simulink model "souk_dual_pipeline_krm"  (R2021a)
settings: Solver=VariableStepAuto  StartTime=0.0  StopTime=10.0  RelTol=1e-3
undefined symbols (not defined in the file): datetime, emio_enet2_tsu_timer_cmp_val_0, posixtime, signal
libraries: xbsIndex_r4 x15746, casper_library_misc x108, casper_library_delays x65, casper_library_reorder x44, xps_library x12
(part 60 of 175)

== system souk_dual_pipeline_krm/p1/synth_input_reorder3/bus_mux ==
  sel : Inport
  d0 : Inport  Port=2
  d1 : Inport  Port=3
  d2 : Inport  Port=4
  d3 : Inport  Port=5
  d4 : Inport  Port=6
  misci : Inport  Port=7
  d_bussify : Subsystem  AncestorBlock=casper_library_flow_control/bus_create  mask(bus_create){inputNum=16}
      mask prompts: inputNum "Number of inputs:"
      mask init:
      | bus_create_init(gcb,...
      |     'inputNum', inputNum);
  dmisc : xbsIndex_r4/Delay  rst=off  infoeditControl=Selection of Reset will increase slice count due to use of real FFs and instead of SRLs  en=off  latency=0  reg_retiming=on  dbl_ovrd=off  block_type=delay
  expand0 : Subsystem  AncestorBlock=casper_library_flow_control/bus_expand  mask(bus_expand){mode=divisions of arbitrary size, outputNum=2, outputWidth=[36;36;36;36;36;36;36;36;36;36;36;36;36;36;36;36], outputBinaryPt=[0  0  0  0  0  0  0  0  0  0  0  0  0  0  0  0], outputArithmeticType=[0  0  0  0  0  0  0  0  0  0  0  0  0  0  0  0], show_format=on, outputToWorkspace=off, variablePrefix=, outputToModelAsWell=on}
      mask prompts: outputNum "Number of outputs:"; outputWidth "Output width:"; outputBinaryPt "Output binary point position:"; outputArithmeticType "Output arithmetic type (ufix=0, fix=1, bool=2):"; show_format "Print format string?"; outputToWorkspace "Output to workspace?"; variablePrefix "Variable name prefix:"; outputToModelAsWell "Output to model as well?"
      mask help:
      | Expands a 'bus' made using a bus_create or Xilinx
      | concat block.
      | The input will be divided into the specified number
      | of outputs with the specified arithmetic types.
      | Divisions are made from most significant bit.
      mask init: same as souk_dual_pipeline_krm/bus_expand
      settings: AttributesFormatString=16 outputs: uf36.0,uf36.0,uf36.0,uf36.0,uf36.0,uf36.0,uf36.0,uf36.0,uf36.0,uf36.0,uf36.0,uf36.0,uf36.0,uf36.0,uf36.0,uf36.0,
      mask TypeOptions mode: divisions of equal size | divisions of arbitrary size
      mask Callback mode: %bus_expand_callback();
      mask Callback outputWidth: %bus_expand_callback();
      mask Callback outputToWorkspace: %bus_expand_callback();
  expand1 : Subsystem  AncestorBlock=casper_library_flow_control/bus_expand  mask(bus_expand){mode=divisions of arbitrary size, outputNum=2, outputWidth=[36;36;36;36;36;36;36;36;36;36;36;36;36;36;36;36], outputBinaryPt=[0  0  0  0  0  0  0  0  0  0  0  0  0  0  0  0], outputArithmeticType=[0  0  0  0  0  0  0  0  0  0  0  0  0  0  0  0], show_format=on, outputToWorkspace=off, variablePrefix=, outputToModelAsWell=on}
      mask prompts: outputNum "Number of outputs:"; outputWidth "Output width:"; outputBinaryPt "Output binary point position:"; outputArithmeticType "Output arithmetic type (ufix=0, fix=1, bool=2):"; show_format "Print format string?"; outputToWorkspace "Output to workspace?"; variablePrefix "Variable name prefix:"; outputToModelAsWell "Output to model as well?"
      mask help:
      | Expands a 'bus' made using a bus_create or Xilinx
      | concat block.
      | The input will be divided into the specified number
      | of outputs with the specified arithmetic types.
      | Divisions are made from most significant bit.
      mask init: same as souk_dual_pipeline_krm/bus_expand
      settings: AttributesFormatString=16 outputs: uf36.0,uf36.0,uf36.0,uf36.0,uf36.0,uf36.0,uf36.0,uf36.0,uf36.0,uf36.0,uf36.0,uf36.0,uf36.0,uf36.0,uf36.0,uf36.0,
      mask TypeOptions mode: divisions of equal size | divisions of arbitrary size
      mask Callback mode: %bus_expand_callback();
      mask Callback outputWidth: %bus_expand_callback();
      mask Callback outputToWorkspace: %bus_expand_callback();
  expand2 : Subsystem  AncestorBlock=casper_library_flow_control/bus_expand  mask(bus_expand){mode=divisions of arbitrary size, outputNum=2, outputWidth=[36;36;36;36;36;36;36;36;36;36;36;36;36;36;36;36], outputBinaryPt=[0  0  0  0  0  0  0  0  0  0  0  0  0  0  0  0], outputArithmeticType=[0  0  0  0  0  0  0  0  0  0  0  0  0  0  0  0], show_format=on, outputToWorkspace=off, variablePrefix=, outputToModelAsWell=on}
      mask prompts: outputNum "Number of outputs:"; outputWidth "Output width:"; outputBinaryPt "Output binary point position:"; outputArithmeticType "Output arithmetic type (ufix=0, fix=1, bool=2):"; show_format "Print format string?"; outputToWorkspace "Output to workspace?"; variablePrefix "Variable name prefix:"; outputToModelAsWell "Output to model as well?"
      mask help:
      | Expands a 'bus' made using a bus_create or Xilinx
      | concat block.
      | The input will be divided into the specified number
      | of outputs with the specified arithmetic types.
      | Divisions are made from most significant bit.
      mask init: same as souk_dual_pipeline_krm/bus_expand
      settings: AttributesFormatString=16 outputs: uf36.0,uf36.0,uf36.0,uf36.0,uf36.0,uf36.0,uf36.0,uf36.0,uf36.0,uf36.0,uf36.0,uf36.0,uf36.0,uf36.0,uf36.0,uf36.0,
      mask TypeOptions mode: divisions of equal size | divisions of arbitrary size
      mask Callback mode: %bus_expand_callback();
      mask Callback outputWidth: %bus_expand_callback();
      mask Callback outputToWorkspace: %bus_expand_callback();
  expand3 : Subsystem  AncestorBlock=casper_library_flow_control/bus_expand  mask(bus_expand){mode=divisions of arbitrary size, outputNum=2, outputWidth=[36;36;36;36;36;36;36;36;36;36;36;36;36;36;36;36], outputBinaryPt=[0  0  0  0  0  0  0  0  0  0  0  0  0  0  0  0], outputArithmeticType=[0  0  0  0  0  0  0  0  0  0  0  0  0  0  0  0], show_format=on, outputToWorkspace=off, variablePrefix=, outputToModelAsWell=on}
      mask prompts: outputNum "Number of outputs:"; outputWidth "Output width:"; outputBinaryPt "Output binary point position:"; outputArithmeticType "Output arithmetic type (ufix=0, fix=1, bool=2):"; show_format "Print format string?"; outputToWorkspace "Output to workspace?"; variablePrefix "Variable name prefix:"; outputToModelAsWell "Output to model as well?"
      mask help:
      | Expands a 'bus' made using a bus_create or Xilinx
      | concat block.
      | The input will be divided into the specified number
      | of outputs with the specified arithmetic types.
      | Divisions are made from most significant bit.
      mask init: same as souk_dual_pipeline_krm/bus_expand
      settings: AttributesFormatString=16 outputs: uf36.0,uf36.0,uf36.0,uf36.0,uf36.0,uf36.0,uf36.0,uf36.0,uf36.0,uf36.0,uf36.0,uf36.0,uf36.0,uf36.0,uf36.0,uf36.0,
      mask TypeOptions mode: divisions of equal size | divisions of arbitrary size
      mask Callback mode: %bus_expand_callback();
      mask Callback outputWidth: %bus_expand_callback();
      mask Callback outputToWorkspace: %bus_expand_callback();
  expand4 : Subsystem  AncestorBlock=casper_library_flow_control/bus_expand  mask(bus_expand){mode=divisions of arbitrary size, outputNum=2, outputWidth=[36;36;36;36;36;36;36;36;36;36;36;36;36;36;36;36], outputBinaryPt=[0  0  0  0  0  0  0  0  0  0  0  0  0  0  0  0], outputArithmeticType=[0  0  0  0  0  0  0  0  0  0  0  0  0  0  0  0], show_format=on, outputToWorkspace=off, variablePrefix=, outputToModelAsWell=on}
      mask prompts: outputNum "Number of outputs:"; outputWidth "Output width:"; outputBinaryPt "Output binary point position:"; outputArithmeticType "Output arithmetic type (ufix=0, fix=1, bool=2):"; show_format "Print format string?"; outputToWorkspace "Output to workspace?"; variablePrefix "Variable name prefix:"; outputToModelAsWell "Output to model as well?"
      mask help:
      | Expands a 'bus' made using a bus_create or Xilinx
      | concat block.
      | The input will be divided into the specified number
      | of outputs with the specified arithmetic types.
      | Divisions are made from most significant bit.
      mask init: same as souk_dual_pipeline_krm/bus_expand
      settings: AttributesFormatString=16 outputs: uf36.0,uf36.0,uf36.0,uf36.0,uf36.0,uf36.0,uf36.0,uf36.0,uf36.0,uf36.0,uf36.0,uf36.0,uf36.0,uf36.0,uf36.0,uf36.0,
      mask TypeOptions mode: divisions of equal size | divisions of arbitrary size
      mask Callback mode: %bus_expand_callback();
      mask Callback outputWidth: %bus_expand_callback();
      mask Callback outputToWorkspace: %bus_expand_callback();
  mux{0..15} (16 alike) : xbsIndex_r4/Mux  inputs=5  en=off  latency=0  precision=Full  arith_type=Unsigned  n_bits=16  bin_pt=14  quantization=Truncate  overflow=Wrap  dbl_ovrd=off  block_type=mux
  sel_expand : Subsystem  AncestorBlock=casper_library_flow_control/bus_expand  mask(bus_expand){mode=divisions of equal size, outputNum=16, outputWidth=3, outputBinaryPt=0, outputArithmeticType=0, show_format=on, outputToWorkspace=off, variablePrefix=, outputToModelAsWell=on}
      mask prompts: outputNum "Number of outputs:"; outputWidth "Output width:"; outputBinaryPt "Output binary point position:"; outputArithmeticType "Output arithmetic type (ufix=0, fix=1, bool=2):"; show_format "Print format string?"; outputToWorkspace "Output to workspace?"; variablePrefix "Variable name prefix:"; outputToModelAsWell "Output to model as well?"
      mask help:
      | Expands a 'bus' made using a bus_create or Xilinx
      | concat block.
      | The input will be divided into the specified number
      | of outputs with the specified arithmetic types.
      | Divisions are made from most significant bit.
      mask init: same as souk_dual_pipeline_krm/bus_expand
      settings: AttributesFormatString=16 outputs: uf3.0,uf3.0,uf3.0,uf3.0,uf3.0,uf3.0,uf3.0,uf3.0,uf3.0,uf3.0,uf3.0,uf3.0,uf3.0,uf3.0,uf3.0,uf3.0,
      mask TypeOptions mode: divisions of equal size | divisions of arbitrary size
      mask Callback mode: %bus_expand_callback();
      mask Callback outputWidth: %bus_expand_callback();
      mask Callback outputToWorkspace: %bus_expand_callback();
  out : Outport
  misco : Outport  Port=2
  wires:
  sel/1 -> sel_expand/1(bus_in)
  d0/1 -> expand0/1(bus_in)
  d1/1 -> expand1/1(bus_in)
  d2/1 -> expand2/1(bus_in)
  d3/1 -> expand3/1(bus_in)
  d4/1 -> expand4/1(bus_in)
  sel_expand/1(msb_out16) -> mux0/1
  expand0/1(msb_out16) -> mux0/2
  expand1/1(msb_out16) -> mux0/3
  expand2/1(msb_out16) -> mux0/4
  expand3/1(msb_out16) -> mux0/5
  expand4/1(msb_out16) -> mux0/6
  sel_expand/2(out15) -> mux1/1
  expand0/2(out15) -> mux1/2
  expand1/2(out15) -> mux1/3
  expand2/2(out15) -> mux1/4
  expand3/2(out15) -> mux1/5
  expand4/2(out15) -> mux1/6
  sel_expand/3(out14) -> mux2/1
  expand0/3(out14) -> mux2/2
  expand1/3(out14) -> mux2/3
  expand2/3(out14) -> mux2/4
  expand3/3(out14) -> mux2/5
  expand4/3(out14) -> mux2/6
  sel_expand/4(out13) -> mux3/1
  expand0/4(out13) -> mux3/2
  expand1/4(out13) -> mux3/3
  expand2/4(out13) -> mux3/4
  expand3/4(out13) -> mux3/5
  expand4/4(out13) -> mux3/6
  sel_expand/5(out12) -> mux4/1
  expand0/5(out12) -> mux4/2
  expand1/5(out12) -> mux4/3
  expand2/5(out12) -> mux4/4
  expand3/5(out12) -> mux4/5
  expand4/5(out12) -> mux4/6
  sel_expand/6(out11) -> mux5/1
  expand0/6(out11) -> mux5/2
  expand1/6(out11) -> mux5/3
  expand2/6(out11) -> mux5/4
  expand3/6(out11) -> mux5/5
  expand4/6(out11) -> mux5/6
  sel_expand/7(out10) -> mux6/1
  expand0/7(out10) -> mux6/2
  expand1/7(out10) -> mux6/3
  expand2/7(out10) -> mux6/4
  expand3/7(out10) -> mux6/5
  expand4/7(out10) -> mux6/6
  sel_expand/8(out9) -> mux7/1
  expand0/8(out9) -> mux7/2
  expand1/8(out9) -> mux7/3
  expand2/8(out9) -> mux7/4
  expand3/8(out9) -> mux7/5
  expand4/8(out9) -> mux7/6
  sel_expand/9(out8) -> mux8/1
  expand0/9(out8) -> mux8/2
  expand1/9(out8) -> mux8/3
  expand2/9(out8) -> mux8/4
  expand3/9(out8) -> mux8/5
  expand4/9(out8) -> mux8/6
  sel_expand/10(out7) -> mux9/1
  expand0/10(out7) -> mux9/2
  expand1/10(out7) -> mux9/3
  expand2/10(out7) -> mux9/4
  expand3/10(out7) -> mux9/5
  expand4/10(out7) -> mux9/6
  sel_expand/11(out6) -> mux10/1
  expand0/11(out6) -> mux10/2
  expand1/11(out6) -> mux10/3
  expand2/11(out6) -> mux10/4
  expand3/11(out6) -> mux10/5
  expand4/11(out6) -> mux10/6
  sel_expand/12(out5) -> mux11/1
  expand0/12(out5) -> mux11/2
  expand1/12(out5) -> mux11/3
  expand2/12(out5) -> mux11/4
  expand3/12(out5) -> mux11/5
  expand4/12(out5) -> mux11/6
  sel_expand/13(out4) -> mux12/1
  expand0/13(out4) -> mux12/2
  expand1/13(out4) -> mux12/3
  expand2/13(out4) -> mux12/4
  expand3/13(out4) -> mux12/5
  expand4/13(out4) -> mux12/6
  sel_expand/14(out3) -> mux13/1
  expand0/14(out3) -> mux13/2
  expand1/14(out3) -> mux13/3
  expand2/14(out3) -> mux13/4
  expand3/14(out3) -> mux13/5
  expand4/14(out3) -> mux13/6
  sel_expand/15(out2) -> mux14/1
  expand0/15(out2) -> mux14/2
  expand1/15(out2) -> mux14/3
  expand2/15(out2) -> mux14/4
  expand3/15(out2) -> mux14/5
  expand4/15(out2) -> mux14/6
  sel_expand/16(lsb_out1) -> mux15/1
  expand0/16(lsb_out1) -> mux15/2
  expand1/16(lsb_out1) -> mux15/3
  expand2/16(lsb_out1) -> mux15/4
  expand3/16(lsb_out1) -> mux15/5
  expand4/16(lsb_out1) -> mux15/6
  misci/1 -> dmisc/1
  mux0/1 -> d_bussify/1(in1)
  mux1/1 -> d_bussify/2(in2)
  mux2/1 -> d_bussify/3(in3)
  mux3/1 -> d_bussify/4(in4)
  mux4/1 -> d_bussify/5(in5)
  mux5/1 -> d_bussify/6(in6)
  mux6/1 -> d_bussify/7(in7)
  mux7/1 -> d_bussify/8(in8)
  mux8/1 -> d_bussify/9(in9)
  mux9/1 -> d_bussify/10(in10)
  mux10/1 -> d_bussify/11(in11)
  mux11/1 -> d_bussify/12(in12)
  mux12/1 -> d_bussify/13(in13)
  mux13/1 -> d_bussify/14(in14)
  mux14/1 -> d_bussify/15(in15)
  mux15/1 -> d_bussify/16(in16)
  d_bussify/1(bus_out) -> out/1
  dmisc/1 -> misco/1

== system souk_dual_pipeline_krm/p1/synth_input_reorder3/bus_replicate ==
  in : Inport
  bussify : Subsystem  AncestorBlock=casper_library_flow_control/bus_create  mask(bus_create){inputNum=16}
      mask prompts: inputNum "Number of inputs:"
      mask init:
      | bus_create_init(gcb,...
      |     'inputNum', inputNum);
  out : Outport
  wires:
  in/1 -> bussify/1(in1), bussify/2(in2), bussify/3(in3), bussify/4(in4), bussify/5(in5), bussify/6(in6), bussify/7(in7), bussify/8(in8), bussify/9(in9), bussify/10(in10), bussify/11(in11), bussify/12(in12), bussify/13(in13), bussify/14(in14), bussify/15(in15), bussify/16(in16)
  bussify/1(bus_out) -> out/1

== system souk_dual_pipeline_krm/p1/synth_input_reorder3/bus_replicate1 ==
  in : Inport
  bussify : Subsystem  AncestorBlock=casper_library_flow_control/bus_create  mask(bus_create){inputNum=16}
      mask prompts: inputNum "Number of inputs:"
      mask init:
      | bus_create_init(gcb,...
      |     'inputNum', inputNum);
  out : Outport
  wires:
  bussify/1(bus_out) -> out/1
  in/1 -> bussify/16(in16), bussify/15(in15), bussify/14(in14), bussify/13(in13), bussify/12(in12), bussify/11(in11), bussify/10(in10), bussify/9(in9), bussify/8(in8), bussify/7(in7), bussify/6(in6), bussify/5(in5), bussify/4(in4), bussify/3(in3), bussify/2(in2), bussify/1(in1)

== system souk_dual_pipeline_krm/p1/synth_input_reorder3/bus_replicate2 ==
  in : Inport
  bussify : Subsystem  AncestorBlock=casper_library_flow_control/bus_create  mask(bus_create){inputNum=16}
      mask prompts: inputNum "Number of inputs:"
      mask init:
      | bus_create_init(gcb,...
      |     'inputNum', inputNum);
  out : Outport
  wires:
  in/1 -> bussify/1(in1), bussify/2(in2), bussify/3(in3), bussify/4(in4), bussify/5(in5), bussify/6(in6), bussify/7(in7), bussify/8(in8), bussify/9(in9), bussify/10(in10), bussify/11(in11), bussify/12(in12), bussify/13(in13), bussify/14(in14), bussify/15(in15), bussify/16(in16)
  bussify/1(bus_out) -> out/1

== system souk_dual_pipeline_krm/p1/synth_input_reorder3/bus_replicate3 ==
  in : Inport
  bussify : Subsystem  AncestorBlock=casper_library_flow_control/bus_create  mask(bus_create){inputNum=16}
      mask prompts: inputNum "Number of inputs:"
      mask init:
      | bus_create_init(gcb,...
      |     'inputNum', inputNum);
  out : Outport
  wires:
  bussify/1(bus_out) -> out/1
  in/1 -> bussify/16(in16), bussify/15(in15), bussify/14(in14), bussify/13(in13), bussify/12(in12), bussify/11(in11), bussify/10(in10), bussify/9(in9), bussify/8(in8), bussify/7(in7), bussify/6(in6), bussify/5(in5), bussify/4(in4), bussify/3(in3), bussify/2(in2), bussify/1(in1)

== system souk_dual_pipeline_krm/p1/synth_input_reorder3/map0 ==
  sync : Inport
  din0 : Inport  Port=2
  Constant1 : xbsIndex_r4/Constant  const=1.0  gui_display_data_type=Boolean  arith_type=Boolean  n_bits=16  bin_pt=14  preci_type=Single  exp_width=8  frac_width=24  explicit_period=on  period=1  equ=P=C  opselect=C  inp2=PCIN>>17  opr=+  inp1=P  carry=CIN  dbl_ovrd=off  block_type=constant
  reord : Subsystem  AncestorBlock=casper_library_reorder/reorder  mask(reorder){map=[2^(serial_chan_bits)-1:-1:0], n_bits=0, n_inputs=1, bram_latency=2, map_latency=1, fanout_latency=0, double_buffer=1, bram_map=off, software_controlled=on, use_control_fanout=on, hide_latency=on}
      mask prompts: map "Output Order:"; n_bits "Data width in"; n_inputs "Number of inputs"; bram_latency "BRAM Latency"; map_latency "Map Latency"; fanout_latency "Fanout latency"; double_buffer "Double Buffer"; bram_map "Use BlockRAM for Map"; software_controlled "Use runtime software control"; use_control_fanout "Control fanout of control to multiple iniputs"; hide_latency "EXPERIMENTAL: Hide control latency"
      mask init: same as souk_dual_pipeline_krm/p0/chan_select/2
      settings: AttributesFormatString=order=2
      mask Help: eval('xlWeb(''http://casper.berkeley.edu/wiki/Reorder'')')
  sync_out : Outport
  dout : Outport  Port=2
  wires:
  reord/3(dout0) -> dout/1
  din0/1 -> reord/3(din0)
  reord/1(sync_out) -> sync_out/1
  Constant1/1 -> reord/2(en)
  sync/1 -> reord/1(sync)
  reord/2(valid) -> ?

== system souk_dual_pipeline_krm/p1/synth_input_reorder3/map1 ==
  sync : Inport
  din0 : Inport  Port=2
  Constant1 : xbsIndex_r4/Constant  const=1.0  gui_display_data_type=Boolean  arith_type=Boolean  n_bits=16  bin_pt=14  preci_type=Single  exp_width=8  frac_width=24  explicit_period=on  period=1  equ=P=C  opselect=C  inp2=PCIN>>17  opr=+  inp1=P  carry=CIN  dbl_ovrd=off  block_type=constant
  reord : Subsystem  AncestorBlock=casper_library_reorder/reorder  mask(reorder){map=[2^(serial_chan_bits)-1:-1:0], n_bits=0, n_inputs=1, bram_latency=2, map_latency=1, fanout_latency=0, double_buffer=1, bram_map=off, software_controlled=on, use_control_fanout=on, hide_latency=on}
      mask prompts: map "Output Order:"; n_bits "Data width in"; n_inputs "Number of inputs"; bram_latency "BRAM Latency"; map_latency "Map Latency"; fanout_latency "Fanout latency"; double_buffer "Double Buffer"; bram_map "Use BlockRAM for Map"; software_controlled "Use runtime software control"; use_control_fanout "Control fanout of control to multiple iniputs"; hide_latency "EXPERIMENTAL: Hide control latency"
      mask init: same as souk_dual_pipeline_krm/p0/chan_select/2
      settings: AttributesFormatString=order=2
      mask Help: eval('xlWeb(''http://casper.berkeley.edu/wiki/Reorder'')')
  sync_out : Outport
  dout : Outport  Port=2
  wires:
  reord/2(valid) -> ?
  sync/1 -> reord/1(sync)
  Constant1/1 -> reord/2(en)
  reord/1(sync_out) -> sync_out/1
  din0/1 -> reord/3(din0)
  reord/3(dout0) -> dout/1

== system souk_dual_pipeline_krm/p1/synth_input_reorder3/map10 ==
  sync : Inport
  din0 : Inport  Port=2
  Constant1 : xbsIndex_r4/Constant  const=1.0  gui_display_data_type=Boolean  arith_type=Boolean  n_bits=16  bin_pt=14  preci_type=Single  exp_width=8  frac_width=24  explicit_period=on  period=1  equ=P=C  opselect=C  inp2=PCIN>>17  opr=+  inp1=P  carry=CIN  dbl_ovrd=off  block_type=constant
  reord : Subsystem  AncestorBlock=casper_library_reorder/reorder  mask(reorder){map=[2^(serial_chan_bits)-1:-1:0], n_bits=0, n_inputs=1, bram_latency=2, map_latency=1, fanout_latency=0, double_buffer=1, bram_map=off, software_controlled=on, use_control_fanout=on, hide_latency=on}
      mask prompts: map "Output Order:"; n_bits "Data width in"; n_inputs "Number of inputs"; bram_latency "BRAM Latency"; map_latency "Map Latency"; fanout_latency "Fanout latency"; double_buffer "Double Buffer"; bram_map "Use BlockRAM for Map"; software_controlled "Use runtime software control"; use_control_fanout "Control fanout of control to multiple iniputs"; hide_latency "EXPERIMENTAL: Hide control latency"
      mask init: same as souk_dual_pipeline_krm/p0/chan_select/2
      settings: AttributesFormatString=order=2
      mask Help: eval('xlWeb(''http://casper.berkeley.edu/wiki/Reorder'')')
  sync_out : Outport
  dout : Outport  Port=2
  wires:
  reord/3(dout0) -> dout/1
  din0/1 -> reord/3(din0)
  reord/1(sync_out) -> sync_out/1
  Constant1/1 -> reord/2(en)
  sync/1 -> reord/1(sync)
  reord/2(valid) -> ?

== system souk_dual_pipeline_krm/p1/synth_input_reorder3/map11 ==
  sync : Inport
  din0 : Inport  Port=2
  Constant1 : xbsIndex_r4/Constant  const=1.0  gui_display_data_type=Boolean  arith_type=Boolean  n_bits=16  bin_pt=14  preci_type=Single  exp_width=8  frac_width=24  explicit_period=on  period=1  equ=P=C  opselect=C  inp2=PCIN>>17  opr=+  inp1=P  carry=CIN  dbl_ovrd=off  block_type=constant
  reord : Subsystem  AncestorBlock=casper_library_reorder/reorder  mask(reorder){map=[2^(serial_chan_bits)-1:-1:0], n_bits=0, n_inputs=1, bram_latency=2, map_latency=1, fanout_latency=0, double_buffer=1, bram_map=off, software_controlled=on, use_control_fanout=on, hide_latency=on}
      mask prompts: map "Output Order:"; n_bits "Data width in"; n_inputs "Number of inputs"; bram_latency "BRAM Latency"; map_latency "Map Latency"; fanout_latency "Fanout latency"; double_buffer "Double Buffer"; bram_map "Use BlockRAM for Map"; software_controlled "Use runtime software control"; use_control_fanout "Control fanout of control to multiple iniputs"; hide_latency "EXPERIMENTAL: Hide control latency"
      mask init: same as souk_dual_pipeline_krm/p0/chan_select/2
      settings: AttributesFormatString=order=2
      mask Help: eval('xlWeb(''http://casper.berkeley.edu/wiki/Reorder'')')
  sync_out : Outport
  dout : Outport  Port=2
  wires:
  reord/2(valid) -> ?
  sync/1 -> reord/1(sync)
  Constant1/1 -> reord/2(en)
  reord/1(sync_out) -> sync_out/1
  din0/1 -> reord/3(din0)
  reord/3(dout0) -> dout/1

== system souk_dual_pipeline_krm/p1/synth_input_reorder3/map12 ==
  sync : Inport
  din0 : Inport  Port=2
  Constant1 : xbsIndex_r4/Constant  const=1.0  gui_display_data_type=Boolean  arith_type=Boolean  n_bits=16  bin_pt=14  preci_type=Single  exp_width=8  frac_width=24  explicit_period=on  period=1  equ=P=C  opselect=C  inp2=PCIN>>17  opr=+  inp1=P  carry=CIN  dbl_ovrd=off  block_type=constant
  reord : Subsystem  AncestorBlock=casper_library_reorder/reorder  mask(reorder){map=[2^(serial_chan_bits)-1:-1:0], n_bits=0, n_inputs=1, bram_latency=2, map_latency=1, fanout_latency=0, double_buffer=1, bram_map=off, software_controlled=on, use_control_fanout=on, hide_latency=on}
      mask prompts: map "Output Order:"; n_bits "Data width in"; n_inputs "Number of inputs"; bram_latency "BRAM Latency"; map_latency "Map Latency"; fanout_latency "Fanout latency"; double_buffer "Double Buffer"; bram_map "Use BlockRAM for Map"; software_controlled "Use runtime software control"; use_control_fanout "Control fanout of control to multiple iniputs"; hide_latency "EXPERIMENTAL: Hide control latency"
      mask init: same as souk_dual_pipeline_krm/p0/chan_select/2
      settings: AttributesFormatString=order=2
      mask Help: eval('xlWeb(''http://casper.berkeley.edu/wiki/Reorder'')')
  sync_out : Outport
  dout : Outport  Port=2
  wires:
  reord/3(dout0) -> dout/1
  din0/1 -> reord/3(din0)
  reord/1(sync_out) -> sync_out/1
  Constant1/1 -> reord/2(en)
  sync/1 -> reord/1(sync)
  reord/2(valid) -> ?

== system souk_dual_pipeline_krm/p1/synth_input_reorder3/map13 ==
  sync : Inport
  din0 : Inport  Port=2
  Constant1 : xbsIndex_r4/Constant  const=1.0  gui_display_data_type=Boolean  arith_type=Boolean  n_bits=16  bin_pt=14  preci_type=Single  exp_width=8  frac_width=24  explicit_period=on  period=1  equ=P=C  opselect=C  inp2=PCIN>>17  opr=+  inp1=P  carry=CIN  dbl_ovrd=off  block_type=constant
  reord : Subsystem  AncestorBlock=casper_library_reorder/reorder  mask(reorder){map=[2^(serial_chan_bits)-1:-1:0], n_bits=0, n_inputs=1, bram_latency=2, map_latency=1, fanout_latency=0, double_buffer=1, bram_map=off, software_controlled=on, use_control_fanout=on, hide_latency=on}
      mask prompts: map "Output Order:"; n_bits "Data width in"; n_inputs "Number of inputs"; bram_latency "BRAM Latency"; map_latency "Map Latency"; fanout_latency "Fanout latency"; double_buffer "Double Buffer"; bram_map "Use BlockRAM for Map"; software_controlled "Use runtime software control"; use_control_fanout "Control fanout of control to multiple iniputs"; hide_latency "EXPERIMENTAL: Hide control latency"
      mask init: same as souk_dual_pipeline_krm/p0/chan_select/2
      settings: AttributesFormatString=order=2
      mask Help: eval('xlWeb(''http://casper.berkeley.edu/wiki/Reorder'')')
  sync_out : Outport
  dout : Outport  Port=2
  wires:
  reord/2(valid) -> ?
  sync/1 -> reord/1(sync)
  Constant1/1 -> reord/2(en)
  reord/1(sync_out) -> sync_out/1
  din0/1 -> reord/3(din0)
  reord/3(dout0) -> dout/1

== system souk_dual_pipeline_krm/p1/synth_input_reorder3/map14 ==
  sync : Inport
  din0 : Inport  Port=2
  Constant1 : xbsIndex_r4/Constant  const=1.0  gui_display_data_type=Boolean  arith_type=Boolean  n_bits=16  bin_pt=14  preci_type=Single  exp_width=8  frac_width=24  explicit_period=on  period=1  equ=P=C  opselect=C  inp2=PCIN>>17  opr=+  inp1=P  carry=CIN  dbl_ovrd=off  block_type=constant
  reord : Subsystem  AncestorBlock=casper_library_reorder/reorder  mask(reorder){map=[2^(serial_chan_bits)-1:-1:0], n_bits=0, n_inputs=1, bram_latency=2, map_latency=1, fanout_latency=0, double_buffer=1, bram_map=off, software_controlled=on, use_control_fanout=on, hide_latency=on}
      mask prompts: map "Output Order:"; n_bits "Data width in"; n_inputs "Number of inputs"; bram_latency "BRAM Latency"; map_latency "Map Latency"; fanout_latency "Fanout latency"; double_buffer "Double Buffer"; bram_map "Use BlockRAM for Map"; software_controlled "Use runtime software control"; use_control_fanout "Control fanout of control to multiple iniputs"; hide_latency "EXPERIMENTAL: Hide control latency"
      mask init: same as souk_dual_pipeline_krm/p0/chan_select/2
      settings: AttributesFormatString=order=2
      mask Help: eval('xlWeb(''http://casper.berkeley.edu/wiki/Reorder'')')
  sync_out : Outport
  dout : Outport  Port=2
  wires:
  reord/2(valid) -> ?
  sync/1 -> reord/1(sync)
  Constant1/1 -> reord/2(en)
  reord/1(sync_out) -> sync_out/1
  din0/1 -> reord/3(din0)
  reord/3(dout0) -> dout/1

== system souk_dual_pipeline_krm/p1/synth_input_reorder3/map15 ==
  sync : Inport
  din0 : Inport  Port=2
  Constant1 : xbsIndex_r4/Constant  const=1.0  gui_display_data_type=Boolean  arith_type=Boolean  n_bits=16  bin_pt=14  preci_type=Single  exp_width=8  frac_width=24  explicit_period=on  period=1  equ=P=C  opselect=C  inp2=PCIN>>17  opr=+  inp1=P  carry=CIN  dbl_ovrd=off  block_type=constant
  reord : Subsystem  AncestorBlock=casper_library_reorder/reorder  mask(reorder){map=[2^(serial_chan_bits)-1:-1:0], n_bits=0, n_inputs=1, bram_latency=2, map_latency=1, fanout_latency=0, double_buffer=1, bram_map=off, software_controlled=on, use_control_fanout=on, hide_latency=on}
      mask prompts: map "Output Order:"; n_bits "Data width in"; n_inputs "Number of inputs"; bram_latency "BRAM Latency"; map_latency "Map Latency"; fanout_latency "Fanout latency"; double_buffer "Double Buffer"; bram_map "Use BlockRAM for Map"; software_controlled "Use runtime software control"; use_control_fanout "Control fanout of control to multiple iniputs"; hide_latency "EXPERIMENTAL: Hide control latency"
      mask init: same as souk_dual_pipeline_krm/p0/chan_select/2
      settings: AttributesFormatString=order=2
      mask Help: eval('xlWeb(''http://casper.berkeley.edu/wiki/Reorder'')')
  sync_out : Outport
  dout : Outport  Port=2
  wires:
  reord/3(dout0) -> dout/1
  din0/1 -> reord/3(din0)
  reord/1(sync_out) -> sync_out/1
  Constant1/1 -> reord/2(en)
  sync/1 -> reord/1(sync)
  reord/2(valid) -> ?

== system souk_dual_pipeline_krm/p1/synth_input_reorder3/map2 ==
  sync : Inport
  din0 : Inport  Port=2
  Constant1 : xbsIndex_r4/Constant  const=1.0  gui_display_data_type=Boolean  arith_type=Boolean  n_bits=16  bin_pt=14  preci_type=Single  exp_width=8  frac_width=24  explicit_period=on  period=1  equ=P=C  opselect=C  inp2=PCIN>>17  opr=+  inp1=P  carry=CIN  dbl_ovrd=off  block_type=constant
  reord : Subsystem  AncestorBlock=casper_library_reorder/reorder  mask(reorder){map=[2^(serial_chan_bits)-1:-1:0], n_bits=0, n_inputs=1, bram_latency=2, map_latency=1, fanout_latency=0, double_buffer=1, bram_map=off, software_controlled=on, use_control_fanout=on, hide_latency=on}
      mask prompts: map "Output Order:"; n_bits "Data width in"; n_inputs "Number of inputs"; bram_latency "BRAM Latency"; map_latency "Map Latency"; fanout_latency "Fanout latency"; double_buffer "Double Buffer"; bram_map "Use BlockRAM for Map"; software_controlled "Use runtime software control"; use_control_fanout "Control fanout of control to multiple iniputs"; hide_latency "EXPERIMENTAL: Hide control latency"
      mask init: same as souk_dual_pipeline_krm/p0/chan_select/2
      settings: AttributesFormatString=order=2
      mask Help: eval('xlWeb(''http://casper.berkeley.edu/wiki/Reorder'')')
  sync_out : Outport
  dout : Outport  Port=2
  wires:
  reord/2(valid) -> ?
  sync/1 -> reord/1(sync)
  Constant1/1 -> reord/2(en)
  reord/1(sync_out) -> sync_out/1
  din0/1 -> reord/3(din0)
  reord/3(dout0) -> dout/1

== system souk_dual_pipeline_krm/p1/synth_input_reorder3/map3 ==
  sync : Inport
  din0 : Inport  Port=2
  Constant1 : xbsIndex_r4/Constant  const=1.0  gui_display_data_type=Boolean  arith_type=Boolean  n_bits=16  bin_pt=14  preci_type=Single  exp_width=8  frac_width=24  explicit_period=on  period=1  equ=P=C  opselect=C  inp2=PCIN>>17  opr=+  inp1=P  carry=CIN  dbl_ovrd=off  block_type=constant
  reord : Subsystem  AncestorBlock=casper_library_reorder/reorder  mask(reorder){map=[2^(serial_chan_bits)-1:-1:0], n_bits=0, n_inputs=1, bram_latency=2, map_latency=1, fanout_latency=0, double_buffer=1, bram_map=off, software_controlled=on, use_control_fanout=on, hide_latency=on}
      mask prompts: map "Output Order:"; n_bits "Data width in"; n_inputs "Number of inputs"; bram_latency "BRAM Latency"; map_latency "Map Latency"; fanout_latency "Fanout latency"; double_buffer "Double Buffer"; bram_map "Use BlockRAM for Map"; software_controlled "Use runtime software control"; use_control_fanout "Control fanout of control to multiple iniputs"; hide_latency "EXPERIMENTAL: Hide control latency"
      mask init: same as souk_dual_pipeline_krm/p0/chan_select/2
      settings: AttributesFormatString=order=2
      mask Help: eval('xlWeb(''http://casper.berkeley.edu/wiki/Reorder'')')
  sync_out : Outport
  dout : Outport  Port=2
  wires:
  reord/3(dout0) -> dout/1
  din0/1 -> reord/3(din0)
  reord/1(sync_out) -> sync_out/1
  Constant1/1 -> reord/2(en)
  sync/1 -> reord/1(sync)
  reord/2(valid) -> ?

== system souk_dual_pipeline_krm/p1/synth_input_reorder3/map4 ==
  sync : Inport
  din0 : Inport  Port=2
  Constant1 : xbsIndex_r4/Constant  const=1.0  gui_display_data_type=Boolean  arith_type=Boolean  n_bits=16  bin_pt=14  preci_type=Single  exp_width=8  frac_width=24  explicit_period=on  period=1  equ=P=C  opselect=C  inp2=PCIN>>17  opr=+  inp1=P  carry=CIN  dbl_ovrd=off  block_type=constant
  reord : Subsystem  AncestorBlock=casper_library_reorder/reorder  mask(reorder){map=[2^(serial_chan_bits)-1:-1:0], n_bits=0, n_inputs=1, bram_latency=2, map_latency=1, fanout_latency=0, double_buffer=1, bram_map=off, software_controlled=on, use_control_fanout=on, hide_latency=on}
      mask prompts: map "Output Order:"; n_bits "Data width in"; n_inputs "Number of inputs"; bram_latency "BRAM Latency"; map_latency "Map Latency"; fanout_latency "Fanout latency"; double_buffer "Double Buffer"; bram_map "Use BlockRAM for Map"; software_controlled "Use runtime software control"; use_control_fanout "Control fanout of control to multiple iniputs"; hide_latency "EXPERIMENTAL: Hide control latency"
      mask init: same as souk_dual_pipeline_krm/p0/chan_select/2
      settings: AttributesFormatString=order=2
      mask Help: eval('xlWeb(''http://casper.berkeley.edu/wiki/Reorder'')')
  sync_out : Outport
  dout : Outport  Port=2
  wires:
  reord/2(valid) -> ?
  sync/1 -> reord/1(sync)
  Constant1/1 -> reord/2(en)
  reord/1(sync_out) -> sync_out/1
  din0/1 -> reord/3(din0)
  reord/3(dout0) -> dout/1

== system souk_dual_pipeline_krm/p1/synth_input_reorder3/map5 ==
  sync : Inport
  din0 : Inport  Port=2
  Constant1 : xbsIndex_r4/Constant  const=1.0  gui_display_data_type=Boolean  arith_type=Boolean  n_bits=16  bin_pt=14  preci_type=Single  exp_width=8  frac_width=24  explicit_period=on  period=1  equ=P=C  opselect=C  inp2=PCIN>>17  opr=+  inp1=P  carry=CIN  dbl_ovrd=off  block_type=constant
  reord : Subsystem  AncestorBlock=casper_library_reorder/reorder  mask(reorder){map=[2^(serial_chan_bits)-1:-1:0], n_bits=0, n_inputs=1, bram_latency=2, map_latency=1, fanout_latency=0, double_buffer=1, bram_map=off, software_controlled=on, use_control_fanout=on, hide_latency=on}
      mask prompts: map "Output Order:"; n_bits "Data width in"; n_inputs "Number of inputs"; bram_latency "BRAM Latency"; map_latency "Map Latency"; fanout_latency "Fanout latency"; double_buffer "Double Buffer"; bram_map "Use BlockRAM for Map"; software_controlled "Use runtime software control"; use_control_fanout "Control fanout of control to multiple iniputs"; hide_latency "EXPERIMENTAL: Hide control latency"
      mask init: same as souk_dual_pipeline_krm/p0/chan_select/2
      settings: AttributesFormatString=order=2
      mask Help: eval('xlWeb(''http://casper.berkeley.edu/wiki/Reorder'')')
  sync_out : Outport
  dout : Outport  Port=2
  wires:
  reord/3(dout0) -> dout/1
  din0/1 -> reord/3(din0)
  reord/1(sync_out) -> sync_out/1
  Constant1/1 -> reord/2(en)
  sync/1 -> reord/1(sync)
  reord/2(valid) -> ?

== system souk_dual_pipeline_krm/p1/synth_input_reorder3/map6 ==
  sync : Inport
  din0 : Inport  Port=2
  Constant1 : xbsIndex_r4/Constant  const=1.0  gui_display_data_type=Boolean  arith_type=Boolean  n_bits=16  bin_pt=14  preci_type=Single  exp_width=8  frac_width=24  explicit_period=on  period=1  equ=P=C  opselect=C  inp2=PCIN>>17  opr=+  inp1=P  carry=CIN  dbl_ovrd=off  block_type=constant
  reord : Subsystem  AncestorBlock=casper_library_reorder/reorder  mask(reorder){map=[2^(serial_chan_bits)-1:-1:0], n_bits=0, n_inputs=1, bram_latency=2, map_latency=1, fanout_latency=0, double_buffer=1, bram_map=off, software_controlled=on, use_control_fanout=on, hide_latency=on}
      mask prompts: map "Output Order:"; n_bits "Data width in"; n_inputs "Number of inputs"; bram_latency "BRAM Latency"; map_latency "Map Latency"; fanout_latency "Fanout latency"; double_buffer "Double Buffer"; bram_map "Use BlockRAM for Map"; software_controlled "Use runtime software control"; use_control_fanout "Control fanout of control to multiple iniputs"; hide_latency "EXPERIMENTAL: Hide control latency"
      mask init: same as souk_dual_pipeline_krm/p0/chan_select/2
      settings: AttributesFormatString=order=2
      mask Help: eval('xlWeb(''http://casper.berkeley.edu/wiki/Reorder'')')
  sync_out : Outport
  dout : Outport  Port=2
  wires:
  reord/3(dout0) -> dout/1
  din0/1 -> reord/3(din0)
  reord/1(sync_out) -> sync_out/1
  Constant1/1 -> reord/2(en)
  sync/1 -> reord/1(sync)
  reord/2(valid) -> ?

== system souk_dual_pipeline_krm/p1/synth_input_reorder3/map7 ==
  sync : Inport
  din0 : Inport  Port=2
  Constant1 : xbsIndex_r4/Constant  const=1.0  gui_display_data_type=Boolean  arith_type=Boolean  n_bits=16  bin_pt=14  preci_type=Single  exp_width=8  frac_width=24  explicit_period=on  period=1  equ=P=C  opselect=C  inp2=PCIN>>17  opr=+  inp1=P  carry=CIN  dbl_ovrd=off  block_type=constant
  reord : Subsystem  AncestorBlock=casper_library_reorder/reorder  mask(reorder){map=[2^(serial_chan_bits)-1:-1:0], n_bits=0, n_inputs=1, bram_latency=2, map_latency=1, fanout_latency=0, double_buffer=1, bram_map=off, software_controlled=on, use_control_fanout=on, hide_latency=on}
      mask prompts: map "Output Order:"; n_bits "Data width in"; n_inputs "Number of inputs"; bram_latency "BRAM Latency"; map_latency "Map Latency"; fanout_latency "Fanout latency"; double_buffer "Double Buffer"; bram_map "Use BlockRAM for Map"; software_controlled "Use runtime software control"; use_control_fanout "Control fanout of control to multiple iniputs"; hide_latency "EXPERIMENTAL: Hide control latency"
      mask init: same as souk_dual_pipeline_krm/p0/chan_select/2
      settings: AttributesFormatString=order=2
      mask Help: eval('xlWeb(''http://casper.berkeley.edu/wiki/Reorder'')')
  sync_out : Outport
  dout : Outport  Port=2
  wires:
  reord/2(valid) -> ?
  sync/1 -> reord/1(sync)
  Constant1/1 -> reord/2(en)
  reord/1(sync_out) -> sync_out/1
  din0/1 -> reord/3(din0)
  reord/3(dout0) -> dout/1

== system souk_dual_pipeline_krm/p1/synth_input_reorder3/map8 ==
  sync : Inport
  din0 : Inport  Port=2
  Constant1 : xbsIndex_r4/Constant  const=1.0  gui_display_data_type=Boolean  arith_type=Boolean  n_bits=16  bin_pt=14  preci_type=Single  exp_width=8  frac_width=24  explicit_period=on  period=1  equ=P=C  opselect=C  inp2=PCIN>>17  opr=+  inp1=P  carry=CIN  dbl_ovrd=off  block_type=constant
  reord : Subsystem  AncestorBlock=casper_library_reorder/reorder  mask(reorder){map=[2^(serial_chan_bits)-1:-1:0], n_bits=0, n_inputs=1, bram_latency=2, map_latency=1, fanout_latency=0, double_buffer=1, bram_map=off, software_controlled=on, use_control_fanout=on, hide_latency=on}
      mask prompts: map "Output Order:"; n_bits "Data width in"; n_inputs "Number of inputs"; bram_latency "BRAM Latency"; map_latency "Map Latency"; fanout_latency "Fanout latency"; double_buffer "Double Buffer"; bram_map "Use BlockRAM for Map"; software_controlled "Use runtime software control"; use_control_fanout "Control fanout of control to multiple iniputs"; hide_latency "EXPERIMENTAL: Hide control latency"
      mask init: same as souk_dual_pipeline_krm/p0/chan_select/2
      settings: AttributesFormatString=order=2
      mask Help: eval('xlWeb(''http://casper.berkeley.edu/wiki/Reorder'')')
  sync_out : Outport
  dout : Outport  Port=2
  wires:
  reord/2(valid) -> ?
  sync/1 -> reord/1(sync)
  Constant1/1 -> reord/2(en)
  reord/1(sync_out) -> sync_out/1
  din0/1 -> reord/3(din0)
  reord/3(dout0) -> dout/1

== system souk_dual_pipeline_krm/p1/synth_input_reorder3/map9 ==
  sync : Inport
  din0 : Inport  Port=2
  Constant1 : xbsIndex_r4/Constant  const=1.0  gui_display_data_type=Boolean  arith_type=Boolean  n_bits=16  bin_pt=14  preci_type=Single  exp_width=8  frac_width=24  explicit_period=on  period=1  equ=P=C  opselect=C  inp2=PCIN>>17  opr=+  inp1=P  carry=CIN  dbl_ovrd=off  block_type=constant
  reord : Subsystem  AncestorBlock=casper_library_reorder/reorder  mask(reorder){map=[2^(serial_chan_bits)-1:-1:0], n_bits=0, n_inputs=1, bram_latency=2, map_latency=1, fanout_latency=0, double_buffer=1, bram_map=off, software_controlled=on, use_control_fanout=on, hide_latency=on}
      mask prompts: map "Output Order:"; n_bits "Data width in"; n_inputs "Number of inputs"; bram_latency "BRAM Latency"; map_latency "Map Latency"; fanout_latency "Fanout latency"; double_buffer "Double Buffer"; bram_map "Use BlockRAM for Map"; software_controlled "Use runtime software control"; use_control_fanout "Control fanout of control to multiple iniputs"; hide_latency "EXPERIMENTAL: Hide control latency"
      mask init: same as souk_dual_pipeline_krm/p0/chan_select/2
      settings: AttributesFormatString=order=2
      mask Help: eval('xlWeb(''http://casper.berkeley.edu/wiki/Reorder'')')
  sync_out : Outport
  dout : Outport  Port=2
  wires:
  reord/3(dout0) -> dout/1
  din0/1 -> reord/3(din0)
  reord/1(sync_out) -> sync_out/1
  Constant1/1 -> reord/2(en)
  sync/1 -> reord/1(sync)
  reord/2(valid) -> ?

== system souk_dual_pipeline_krm/p1/synth_input_reorder3/munge1 ==
  din : Inport
  join : Subsystem  AncestorBlock=casper_library_flow_control/bus_create  mask(bus_create){inputNum=16}
      mask prompts: inputNum "Number of inputs:"
      mask init:
      | bus_create_init(gcb,...
      |     'inputNum', inputNum);
  reinterpret : xbsIndex_r4/Reinterpret  force_arith_type=on  arith_type=Unsigned  force_bin_pt=on  bin_pt=0  block_type=reinterpret
  reinterpret_out : xbsIndex_r4/Reinterpret  force_arith_type=on  arith_type=Unsigned  force_bin_pt=on  bin_pt=0  block_type=reinterpret
  split : Subsystem  AncestorBlock=casper_library_flow_control/bus_expand  mask(bus_expand){mode=divisions of arbitrary size, outputNum=16, outputWidth=[36;36;36;36;36;36;36;36;36;36;36;36;36;36;36;36], outputBinaryPt=[0 0 0 0 0 0 0 0 0 0 0 0 0 0 0 0], outputArithmeticType=[0 0 0 0 0 0 0 0 0 0 0 0 0 0 0 0], show_format=off, outputToWorkspace=off, variablePrefix=out, outputToModelAsWell=on}
      mask prompts: outputNum "Number of outputs:"; outputWidth "Output width:"; outputBinaryPt "Output binary point position:"; outputArithmeticType "Output arithmetic type (ufix=0, fix=1, bool=2):"; show_format "Print format string?"; outputToWorkspace "Output to workspace?"; variablePrefix "Variable name prefix:"; outputToModelAsWell "Output to model as well?"
      mask help:
      | Expands a 'bus' made using a bus_create or Xilinx
      | concat block.
      | The input will be divided into the specified number
      | of outputs with the specified arithmetic types.
      | Divisions are made from most significant bit.
      mask init: same as souk_dual_pipeline_krm/bus_expand
      settings: AttributesFormatString=16 outputs
      mask TypeOptions mode: divisions of equal size | divisions of arbitrary size
      mask Callback mode: %bus_expand_callback();
      mask Callback outputWidth: %bus_expand_callback();
      mask Callback outputToWorkspace: %bus_expand_callback();
  dout : Outport
  wires:
  reinterpret_out/1 -> dout/1
  din/1 -> reinterpret/1
  reinterpret/1 -> split/1(bus_in)
  join/1(bus_out) -> reinterpret_out/1
  split/1(msb_out16) -> join/1(in1)
  split/3(out14) -> join/2(in2)
  split/5(out12) -> join/3(in3)
  split/7(out10) -> join/4(in4)
  split/9(out8) -> join/5(in5)
  split/11(out6) -> join/6(in6)
  split/13(out4) -> join/7(in7)
  split/15(out2) -> join/8(in8)
  split/2(out15) -> join/9(in9)
  split/4(out13) -> join/10(in10)
  split/6(out11) -> join/11(in11)
  split/8(out9) -> join/12(in12)
  split/10(out7) -> join/13(in13)
  split/12(out5) -> join/14(in14)
  split/14(out3) -> join/15(in15)
  split/16(lsb_out1) -> join/16(in16)
